simulink model "WDS2"  (R2022b)
settings: Solver=VariableStepAuto  StartTime=0.0  StopTime=86400  RelTol=0.034
libraries: sh_lib x46, nesl_utility x16, fl_lib x12, SignalEditorBlockLib x3
(part 2 of 2)

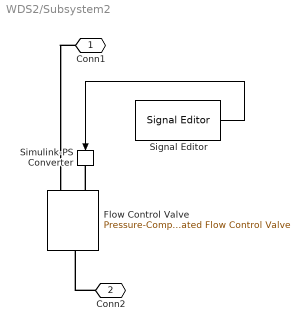
== system WDS2/Subsystem2 ==
  Flow Control Valve : sh_lib/Valves/Flow Control Valves/Pressure-Compensated Flow Control Valve  Tag=Factory Generic  mdl_type=1  area_max=0.86e-4 m^2  opening_max=0.016 m  opening_tab="[  -0.002 0 0.005 0.015 ] m"  area_tab="[  1e-12 4e-12 1e-05 1.02e-05 ] m^2"  interp_method=1  extrap_method=1  pr_dif=6e+05 Pa  reg_range=5e+04 Pa  C_d=0.7  x_0=0 m  A_leak=1e-12 m^2  lam_spec=1  B_lam=0.999  Re_cr=12
      settings: InternalSimscapePortConfiguration="{\"Bottom\":[],\"Left\":[{\"id\":\"C\",\"label\":\"C\",\"type\":\"input\"},{\"id\":\"A\",\"label\":\"A\",\"type\":\"foundation.hydraulic.hydraulic\"}],\"Right\":[{\"id\":\"B\",\"label\":\"B\",\"type\":\"foundation.hydraulic.hydraulic\"}],\"Top\":[]}"
  Signal Editor : SignalEditorBlockLib/Signal Editor  FileName=/Users/philip/Desktop/untitled folder/Untitled.mat  ActiveScenario=Scenario  ActiveSignal=Signal 1  IsBus=off  OutputBusObjectStr=Bus: BusObject  SampleTime=0  Interpolate=off  ZeroCross=off  OutputAfterFinalValue=Setting to zero  Unit=inherit  PreserveSignalName=on
  Simulink-PS Converter : nesl_utility/Simulink-PS Converter  PhysicalDomain=network_engine_domain  SubClassName=ps_input  LeftPortType=input  RightPortType=output  PseudoPeriodic=off  Frequencies=[]  NoiseDistribution=none  NoiseParameters=[]  Unit=1  AffineConversion=off  FilteringAndDerivatives=provide  SimscapeFilterOrder=1  InputFilterTimeConstant=0.001  UdotUserProvided=0
  Conn1 : PMIOPort  Side=Left
  Conn2 : PMIOPort  Port=2  Side=Right
  wires:
  Signal Editor/1 -> Simulink-PS Converter/1
  connections:
  Conn1/RConn1 -- Flow Control Valve/LConn2
  Conn2/RConn1 -- Flow Control Valve/RConn1
  Flow Control Valve/LConn1 -- Simulink-PS Converter/RConn1

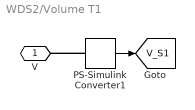
== system WDS2/Volume T1 ==
  PS-Simulink Converter1 : nesl_utility/PS-Simulink Converter  PhysicalDomain=network_engine_domain  SubClassName=ps_output  LeftPortType=input  RightPortType=output  PseudoPeriodic=off  Frequencies=[]  VectorFormat=1-D array  Unit=1  AffineConversion=off
  V : PMIOPort  Side=Left
  tag scope: V_S1=global
  wires:
  PS-Simulink Converter1/1 -> [V_S1]
  connections:
  PS-Simulink Converter1/LConn1 -- V/RConn1

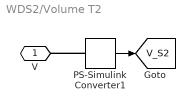
== system WDS2/Volume T2 ==
  PS-Simulink Converter1 : nesl_utility/PS-Simulink Converter  PhysicalDomain=network_engine_domain  SubClassName=ps_output  LeftPortType=input  RightPortType=output  PseudoPeriodic=off  Frequencies=[]  VectorFormat=1-D array  Unit=1  AffineConversion=off
  V : PMIOPort  Side=Left
  tag scope: V_S2=global
  wires:
  PS-Simulink Converter1/1 -> [V_S2]
  connections:
  PS-Simulink Converter1/LConn1 -- V/RConn1

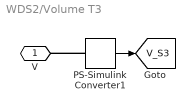
== system WDS2/Volume T3 ==
  PS-Simulink Converter1 : nesl_utility/PS-Simulink Converter  PhysicalDomain=network_engine_domain  SubClassName=ps_output  LeftPortType=input  RightPortType=output  PseudoPeriodic=off  Frequencies=[]  VectorFormat=1-D array  Unit=1  AffineConversion=off
  V : PMIOPort  Side=Left
  tag scope: V_S3=global
  wires:
  PS-Simulink Converter1/1 -> [V_S3]
  connections:
  PS-Simulink Converter1/LConn1 -- V/RConn1

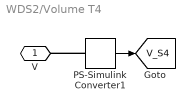
== system WDS2/Volume T4 ==
  PS-Simulink Converter1 : nesl_utility/PS-Simulink Converter  PhysicalDomain=network_engine_domain  SubClassName=ps_output  LeftPortType=input  RightPortType=output  PseudoPeriodic=off  Frequencies=[]  VectorFormat=1-D array  Unit=1  AffineConversion=off
  V : PMIOPort  Side=Left
  tag scope: V_S4=global
  wires:
  PS-Simulink Converter1/1 -> [V_S4]
  connections:
  PS-Simulink Converter1/LConn1 -- V/RConn1

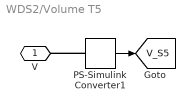
== system WDS2/Volume T5 ==
  PS-Simulink Converter1 : nesl_utility/PS-Simulink Converter  PhysicalDomain=network_engine_domain  SubClassName=ps_output  LeftPortType=input  RightPortType=output  PseudoPeriodic=off  Frequencies=[]  VectorFormat=1-D array  Unit=1  AffineConversion=off
  V : PMIOPort  Side=Left
  tag scope: V_S5=global
  wires:
  PS-Simulink Converter1/1 -> [V_S5]
  connections:
  PS-Simulink Converter1/LConn1 -- V/RConn1

== system WDS2/Volume T6 ==
  PS-Simulink Converter1 : nesl_utility/PS-Simulink Converter  PhysicalDomain=network_engine_domain  SubClassName=ps_output  LeftPortType=input  RightPortType=output  PseudoPeriodic=off  Frequencies=[]  VectorFormat=1-D array  Unit=1  AffineConversion=off
  V : PMIOPort  Side=Left
  tag scope: V_S6=global
  wires:
  PS-Simulink Converter1/1 -> [V_S6]
  connections:
  PS-Simulink Converter1/LConn1 -- V/RConn1
